simulink model "untitled"  (R2021b)
settings: Solver=VariableStepAuto  StartTime=0.0  StopTime=0.1  RelTol=1e-3
settings Model: Creator=Dajun  LastModifiedBy=Dajun

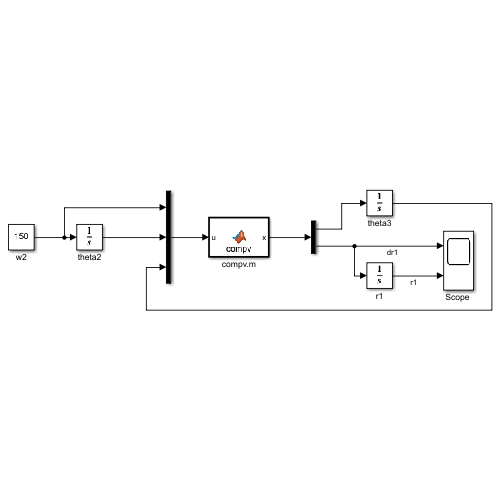
[thumbnail: Simulink's stored preview of the top-level diagram]
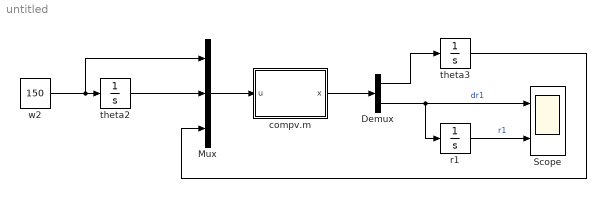
== system untitled ==
  Demux : Demux  Outputs=2
  Mux : Mux  Inputs=3
  "Scope " : Scope  NumInputPorts=2
  compv.m : MATLAB Function  TreatAsAtomicUnit=on
  r1 : Integrator  InitialCondition=70
  theta2 : Integrator
  theta3 : Integrator
  w2 : Constant  Value=150  SampleTime=Inf
  wires:
  Demux/2 -> r1/1, "Scope "/1  "dr1"
  r1/1 -> "Scope "/2  "r1"
  Demux/1 -> theta3/1
  compv.m/1(x) -> Demux/1
  Mux/1 -> compv.m/1(u)
  theta2/1 -> Mux/2
  w2/1 -> Mux/1, theta2/1
  theta3/1 -> Mux/3

== matlab function untitled/compv.m ==
  data: u input; x output
function x  = compv(u)
%u(1) = w2
%u(2) = theta2
%u(3) = theta3
a=zeros(2,2);
b=zeros(2,1);
x=zeros(2,1);
r2 = 15;
r3 = 55 ; %连杆 2、 3 的长度
a=[r3*sin(u(3)) 1; -r3*cos(u(3)) 0]; %求解运动学方程
b=[-r2*u(1)*sin(u(2)); r2*u(1)*cos(u(2))];
x=inv(a)*b;
